simulink model "ReqsGroundTruth"  (R2021b)
settings: Solver=FixedStepAuto  StartTime=0.0  StopTime=stopTime  RelTol=1e-3
model workspace (MAT data in the model file):
  firstWarning = 1
  originalScenarioChecksum = '114339432DE22364D47BB28FC96DC10C'
undefined symbols (not defined in the file): Acceleration, ActorID, AngularVelocity, DefaultGear, DEND_B, DEND_S, DEND_T, LF, LR, MAX_BRAKE, MAX_STEER, MAX_TORQUE, MCAR, MIN_BRAKE, MIN_STEER, MIN_TORQUE, NUMD_B, NUMD_S, NUMD_T, Pitch, Position, R, Roll, RRdamp, scenario, sigbuilder_block, STEER_RATIO, stopSign_ID, Tdead, TL_ID, TrackWidth, Ts, ts, Vdead, Velocity, X_o, Y_o, Yaw
libraries: sim3dprobsensorlib x2, sim3dcameralib x2, drivingscenarioandsensors x2, simulink x1, mspsensorlib x1, sim3dphyssensorlib x1, autolibshared x1, vehdynlibviscommon x1, vehdynlibsteering x1
settings Model: SimulationMode=software-in-the-loop (sil)  Creator=akshran  LastModifiedBy=akshran
settings OptimizationCC: DefaultParameterBehavior=Inlined  EnhancedBackFolding=on  PassReuseOutputArgsAs=Individual arguments  ZeroExternalMemoryAtStartup=off  ZeroInternalMemoryAtStartup=off  OptimizeBlockOrder=speed  DifferentSizesBufferReuse=on  OptimizationCustomize=off  EfficientTunableParamExpr=on
settings DebuggingCC: ParameterTunabilityLossMsg=error
settings SFSimCC: MATLABDynamicMemAlloc=off
settings RTWCC: Description=Embedded Coder  SystemTargetFile=ert.tlc  TemplateMakefile=ert_default_tmf  BuildConfiguration=Faster Runs  CodeExecutionProfiling=on  CodeProfilingSaveOptions=AllData  TargetLang=C++
settings CodeAppCC: ForceParamTrailComments=on  IgnoreCustomStorageClasses=off  OperatorAnnotations=on  SimulinkDataObjDesc=on  SFDataObjDesc=on  InsertBlockDesc=on
settings ERTTargetCC: TargetLangStandard=C++11 (ISO)  GenerateSampleERTMain=on  CodeInterfacePackaging=C++ class  SupportContinuousTime=on  SupportVariableSizeSignals=on  InlinedParameterPlacement=NonHierarchical  RootIOFormat=Structure reference  ERTCustomFileTemplate=example_file_process.tlc
settings ConfigComp: CovEnable=on  CovScope=ReferencedModels  CovIncludeTopModel=off  CovMetricSettings=dtrzoibwe  CovModelRefEnable=filtered

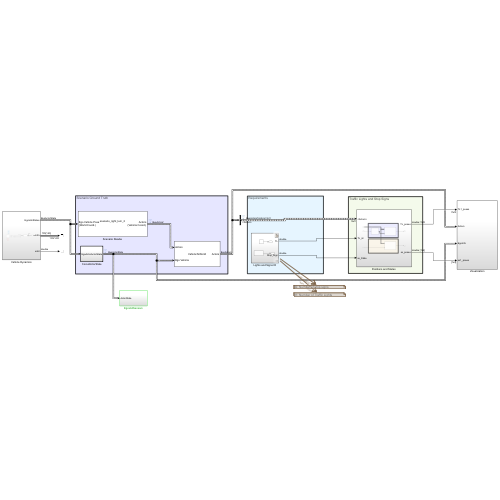
[thumbnail: Simulink's stored preview of the top-level diagram]
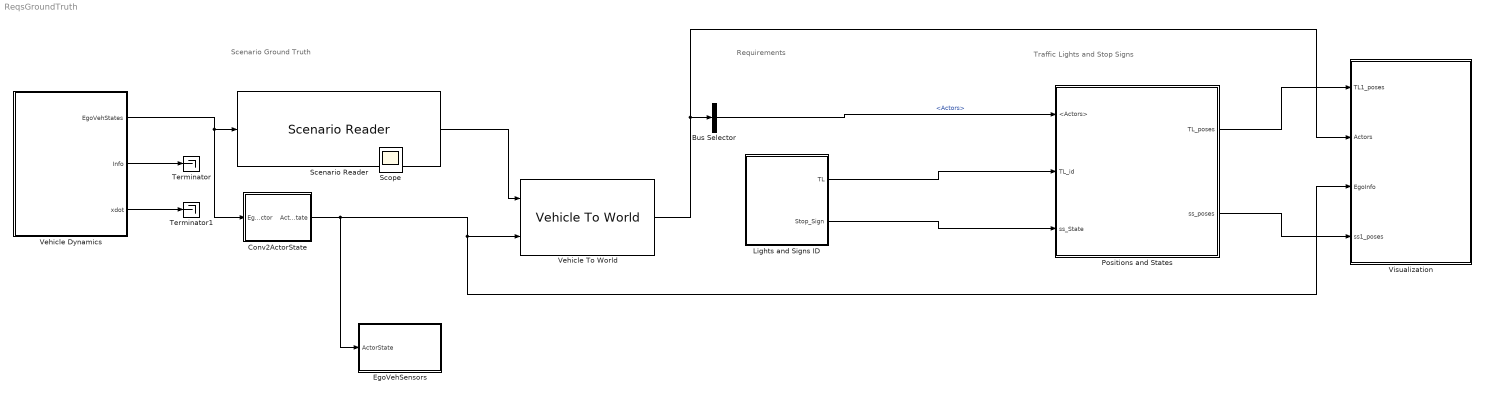
== system ReqsGroundTruth ==
  note: Traffic Lights and Stop Signs
  note: Requirements
  note: Scenario Ground Truth
  Bus Selector : BusSelector  OutputSignals=Actors
  Conv2ActorState : Subsystem  TreatAsAtomicUnit=on
  EgoVehSensors : Subsystem
  Lights and Signs ID : Subsystem
  "Positions and States " : Subsystem
  Scenario Reader : drivingscenarioandsensors/Scenario Reader  ScenarioSource=From file  ScenarioFileName=C:\Users\akshran\MATLAB\Projects\ad2_y1_simulationpkg\scenarios\scenario_right_turn_2.mat  ScenarioVariableName=scenario  OutputCoordinateSystem=Vehicle coordinates  EgoVehicleSource=Input port  EgoVehicleActorID=1  OrientVehiclesOnRoad=on  OutputEgoVehiclePose=on  OutputEgoVehicleState=off  SampleTime=Ts  LaneBoundaryOutput=None  LaneBoundaryDistance=0:0.5:9.5  LaneBoundaryLocation=Center of lane markings  BusNameSource=Auto  BusName=BusActors  BusNumActorsSource=Scenario  BusNumActors=100  BusName2Source=Auto  BusName2=BusLaneBoundaries  BusNumLaneBoundariesSource=Scenario  BusNumLaneBoundaries=10  BusName3Source=Auto  BusName3=BusEgoActor  BusName4Source=Auto  BusName4=BusEgoState  ShowCoordinateLabels=on  SimulateUsing=Interpreted execution
  Terminator : Terminator
  Terminator1 : Terminator
  Vehicle Dynamics : Subsystem
  Vehicle To World : drivingscenarioandsensors/Vehicle To World  BusNameSource=Auto  BusName=BusVehicleToWorldActors  SimulateUsing=Interpreted execution
      settings: SourceProductBaseCode=DR
  Visualization : Subsystem
  Scope : Scope
  wires:
  Vehicle Dynamics/1(EgoVehStates) -> Conv2ActorState/1(EgoActor), Scenario Reader/1
  Scenario Reader/1 -> Vehicle To World/1
  Conv2ActorState/1(ActorState) -> Visualization/3(EgoInfo), Vehicle To World/2, EgoVehSensors/1(ActorState)
  Vehicle To World/1 -> Visualization/2(Actors), Bus Selector/1
  Vehicle Dynamics/2(Info) -> Terminator/1
  Vehicle Dynamics/3(xdot) -> Terminator1/1
  Bus Selector/1 -> "Positions and States "/1(<Actors>)  "<Actors>"
  Lights and Signs ID/1(TL) -> "Positions and States "/2(TL_id)
  Lights and Signs ID/2(Stop_Sign) -> "Positions and States "/3(ss_State)
  "Positions and States "/1(TL_poses) -> Visualization/1(TL1_poses)
  "Positions and States "/2(ss_poses) -> Visualization/4(ss1_poses)

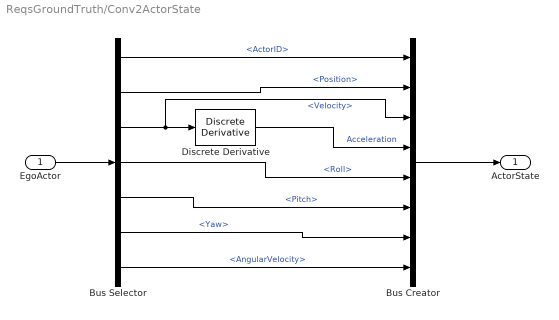
== system ReqsGroundTruth/Conv2ActorState ==
  EgoActor : Inport
  Bus Creator : BusCreator  Inputs=ActorID,Position,Velocity,Acceleration,Roll,Pitch,Yaw,AngularVelocity  OutDataTypeStr=Bus: BusActorState  NonVirtualBus=on
  Bus Selector : BusSelector  OutputSignals=ActorID,Position,Velocity,Roll,Pitch,Yaw,AngularVelocity
  Discrete Derivative : simulink/Discrete/Discrete Derivative  gainval=1.0  ICPrevScaledInput=0.0  OutMin=[]  OutMax=[]  OutDataType=fixdt(1, 16)  OutScaling=2^-10  DoSatur=off
  ActorState : Outport
  wires:
  Bus Selector/3 -> Bus Creator/3, Discrete Derivative/1  "<Velocity>"
  Bus Selector/2 -> Bus Creator/2  "<Position>"
  Bus Selector/7 -> Bus Creator/8  "<AngularVelocity>"
  Discrete Derivative/1 -> Bus Creator/4  "Acceleration"
  Bus Selector/1 -> Bus Creator/1  "<ActorID>"
  Bus Selector/6 -> Bus Creator/7  "<Yaw>"
  Bus Selector/5 -> Bus Creator/6  "<Pitch>"
  Bus Selector/4 -> Bus Creator/5  "<Roll>"
  EgoActor/1 -> Bus Selector/1
  Bus Creator/1 -> ActorState/1

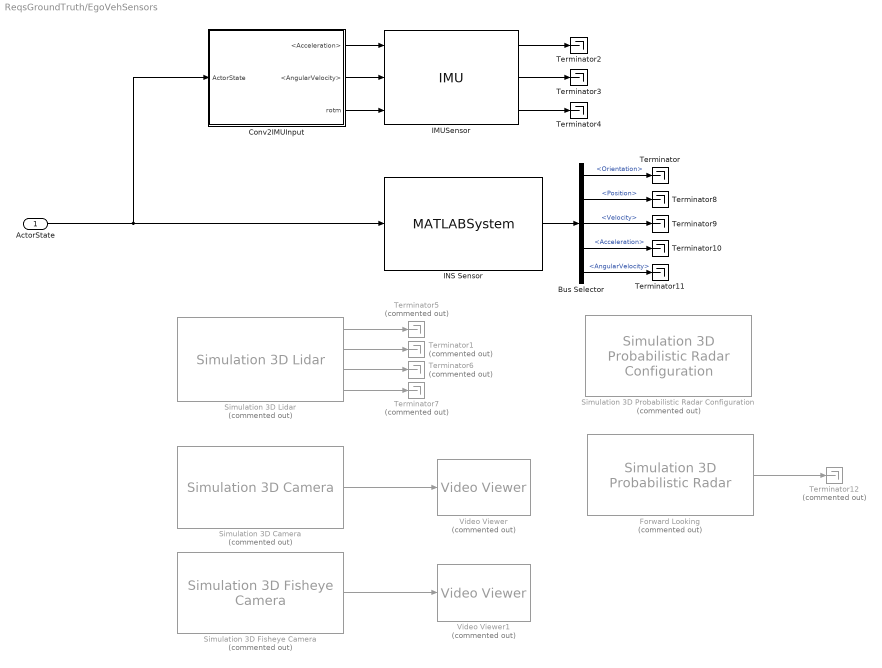
== system ReqsGroundTruth/EgoVehSensors ==
  ActorState : Inport
  Bus Selector : BusSelector  OutputSignals=Orientation,Position,Velocity,Acceleration,AngularVelocity
  Conv2IMUInput : Subsystem  TreatAsAtomicUnit=on
  Forward Looking : sim3dprobsensorlib/Simulation 3D Probabilistic Radar  Priority=1  Commented=on  sensorTag=Sim3dSensor1  sensorId=1  sensorName=Sim3dSensor1  vehTagList={'Scene Origin'}  vehTag=Scene Origin  mountLoc=Origin  offsetFlag=off  tmountOffset=[0, 0, 0]  rmountOffset=[0, 0, 0]  AzimuthResolution=4  ElevationResolution=10  RangeResolution=2.5  RangeRateResolution=0.5  AzimuthBiasFraction=0.1  ElevationBiasFraction=0.1  RangeBiasFraction=0.05  RangeRateBiasFraction=0.05  FieldOfView=[ 45, 5 ]  DetectionRange=[ 1, 150 ]  RangeRateLimits=[ -100, 100 ]  DetectionProbability=0.9  FalseAlarmRate=1e-6  ReferenceRange=100  ReferenceRCS=0  HasElevation=off  HasRangeRate=on  HasNoise=on  HasFalseAlarms=on  InitialSeedSource=Repeatable  InitialSeed=0  MaxNumDetections=50  DetectionCoordinates=Ego Cartesian  SpecifyOutputBusName=off  BusName=BusSimulation3DRadarTruthSensor  SampleTime=-1  mountPoint=[0 0 0]  mountOrientation=[0 0 0]  aMode=3  ID=1
      settings: SourceProductBaseCode=AE,DR,UV,VE
  IMUSensor : mspsensorlib/IMU  DispRefFrame=NED  Temperature=25  MagneticFieldNED=[ 27.5550, -2.4169, -16.0849 ]  MagneticFieldENU=[ -2.4169, 27.5550, 16.0849 ]  SeedDouble=67  SimulateUsing=Interpreted execution  AccelParamsMeasurementRange=Inf  AccelParamsResolution=0  AccelParamsConstantBias=[ 0, 0, 0 ]  AccelParamsAxesMisalignment=[ 0, 0, 0 ]  AccelParamsNoiseDensity=[ 0, 0, 0 ]  AccelParamsBiasInstability=[ 0, 0, 0 ]  AccelParamsRandomWalk=[ 0, 0, 0 ]  AccelParamsTemperatureBias=[ 0, 0, 0 ]  AccelParamsTemperatureScaleFactor=[ 0, 0, 0 ]  GyroParamsMeasurementRange=Inf  GyroParamsResolution=0  GyroParamsConstantBias=[ 0, 0, 0 ]  GyroParamsAxesMisalignment=[ 0, 0, 0 ]  GyroParamsAccelerationBias=[ 0, 0, 0 ]  GyroParamsNoiseDensity=[ 0, 0, 0 ]  GyroParamsBiasInstability=[ 0, 0, 0 ]  GyroParamsRandomWalk=[ 0, 0, 0 ]  GyroParamsTemperatureBias=[ 0, 0, 0 ]  GyroParamsTemperatureScaleFactor=[ 0, 0, 0 ]  MagParamsMeasurementRange=Inf  MagParamsResolution=0  MagParamsConstantBias=[ 0, 0, 0 ]  MagParamsAxesMisalignment=[ 0, 0, 0 ]  MagParamsNoiseDensity=[ 0, 0, 0 ]  MagParamsBiasInstability=[ 0, 0, 0 ]  MagParamsRandomWalk=[ 0, 0, 0 ]  MagParamsTemperatureBias=[ 0, 0, 0 ]  MagParamsTemperatureScaleFactor=[ 0, 0, 0 ]
      settings: SourceProductBaseCode=TF,NV
  INS Sensor : MATLABSystem  System=insSensorBlk  MountingLocation=[ 0, 0, 0 ]  RollAccuracy=0.2  PitchAccuracy=0.2  YawAccuracy=1  PositionAccuracy=[ 1, 1, 1 ]  VelocityAccuracy=0.1  AccelerationAccuracy=0.05  AngularVelocityAccuracy=0.5  PositionErrorFactor=[ 0, 0, 0 ]  OutputBusName1=BusINSMeas  SimulateUsing=Interpreted execution
      mask Type: insSensorBlk
      mask Display:
      | disp('insSensorBlk');
      | port_label('input',1,'ActorStateIn');
      | port_label('output',1,'insMeas');
  Simulation 3D Camera : sim3dcameralib/Simulation 3D Camera  Priority=1  Commented=on  sensorTag=Sim3dSensor2  sensorId=2  sensorName=Sim3dSensor2  vehTagList={'Scene Origin'}  vehTag=Scene Origin  mountLoc=Origin  offsetFlag=off  tmountOffset=[0, 0, 0]  extTmount=off  rmountOffset=[0, 0, 0]  extRmount=off  FocalLength=[1109, 1109]  OpticalCenter=[640, 360]  ImageSize=[720, 1280]  RadialDistortion=[0, 0]  TangentialDistortion=[0, 0]  SensorSkew=0  DepthOutportEnabled=off  SemanticOutportEnabled=off  TransformOutportEnabled=off  SampleTime=-1  mountPoint=[0 0 0]  mountOrientation=[0 0 0]  aMode=3  ID=2
      settings: SourceProductBaseCode=AE,DR,UV,VE
  Simulation 3D Fisheye Camera : sim3dcameralib/Simulation 3D Fisheye Camera  Priority=1  Commented=on  sensorTag=Sim3dSensor3  sensorId=3  sensorName=Sim3dSensor3  vehTagList={'Scene Origin'}  vehTag=Scene Origin  mountLoc=Origin  offsetFlag=off  tmountOffset=[0, 0, 0]  extTmount=off  rmountOffset=[0, 0, 0]  extRmount=off  OpticalCenter=[640, 360]  ImageSize=[720, 1280]  RadialDistortion=[320, 0, 0, 0]  StretchMatrix=[1, 0; 0, 1]  TransformOutportEnabled=off  SampleTime=-1  mountPoint=[0 0 0]  mountOrientation=[0 0 0]  aMode=3  ID=3
      settings: SourceProductBaseCode=AE,DR,UV,VE
  Simulation 3D Lidar : sim3dphyssensorlib/Simulation 3D Lidar  Priority=1  Commented=on  sensorTag=Sim3dSensor4  sensorId=4  sensorName=Sim3dSensor4  vehTagList={'Scene Origin'}  vehTag=Scene Origin  mountLoc=Origin  offsetFlag=off  tmountOffset=[0, 0, 0]  rmountOffset=[0, 0, 0]  DetectionRange=120  RangeResolution=0.002  VerticalFOV=40  VerticalResolution=1.25  HorizontalFOV=360  HorizontalResolution=0.16  DistanceOutportEnabled=on  TransformOutportEnabled=on  SampleTime=0.05  mountPoint=[0 0 0]  mountOrientation=[0 0 0]  aMode=3  ID=4
      settings: SourceProductBaseCode=AE,DR,UV,VE
  Simulation 3D Probabilistic Radar Configuration : sim3dprobsensorlib/Simulation 3D Probabilistic Radar Configuration  Commented=on  RCSactorKeys=[10]  RCSactorProfiles={[10, 10;10, 10]}  RCSdefaultValue=-20  aMode=3
      settings: SourceProductBaseCode=AE,DR,UV,VE
  Terminator{,2..4,8..11} (8 alike) : Terminator
  Terminator{1,5..7,12} (5 alike) : Terminator  Commented=on
  Video Viewer : VideoViewer  Commented=on  FigPos=[1958 858 1025 616]
  Video Viewer1 : VideoViewer  Commented=on  FigPos=[2014 821 1025 616]
  wires:
  ActorState/1 -> INS Sensor/1, Conv2IMUInput/1(ActorState)
  INS Sensor/1 -> Bus Selector/1
  IMUSensor/1 -> Terminator2/1
  IMUSensor/2 -> Terminator3/1
  IMUSensor/3 -> Terminator4/1
  Conv2IMUInput/1(<Acceleration>) -> IMUSensor/1
  Conv2IMUInput/2(<AngularVelocity>) -> IMUSensor/2
  Conv2IMUInput/3(rotm) -> IMUSensor/3
  Simulation 3D Lidar/1 -> Terminator5/1
  Simulation 3D Camera/1 -> Video Viewer/1
  Simulation 3D Lidar/2 -> Terminator1/1
  Simulation 3D Lidar/3 -> Terminator6/1
  Simulation 3D Lidar/4 -> Terminator7/1
  Simulation 3D Fisheye Camera/1 -> Video Viewer1/1
  Bus Selector/1 -> Terminator/1  "<Orientation>"
  Bus Selector/2 -> Terminator8/1  "<Position>"
  Bus Selector/3 -> Terminator9/1  "<Velocity>"
  Bus Selector/4 -> Terminator10/1  "<Acceleration>"
  Bus Selector/5 -> Terminator11/1  "<AngularVelocity>"
  Forward Looking/1 -> Terminator12/1

== system ReqsGroundTruth/Lights and Signs ID ==
  Constant : Constant  Value=TL_ID
  Constant1 : Constant  Value=stopSign_ID
  TL : Outport
  Stop_Sign : Outport  Port=2
  wires:
  Constant/1 -> TL/1
  Constant1/1 -> Stop_Sign/1

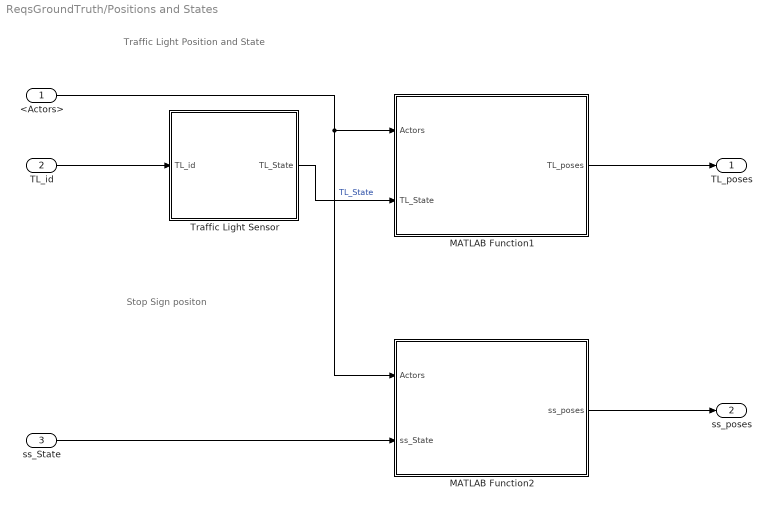
== system ReqsGroundTruth/Positions and States  ==
  note: Stop Sign positon
  note: Traffic Light Position and State
  <Actors> : Inport
  TL_id : Inport  Port=2
  ss_State : Inport  Port=3
  MATLAB Function1 : MATLAB Function  TreatAsAtomicUnit=on
  MATLAB Function2 : MATLAB Function  TreatAsAtomicUnit=on
  Traffic Light Sensor : Subsystem  mask{TrafficLightSensorModeSelection=Cycle}
      mask prompts: TrafficLightSensorModeSelection "Traffic Light Sensor Mode:"
      mask TypeOptions TrafficLightSensorModeSelection: Steady Green | Steady Red | Cycle
      mask DialogControl DescTextVar Prompt: Simulate a traffic light sensor.
  TL_poses : Outport
  ss_poses : Outport  Port=2
  wires:
  <Actors>/1 -> MATLAB Function2/1(Actors), MATLAB Function1/1(Actors)
  ss_State/1 -> MATLAB Function2/2(ss_State)
  TL_id/1 -> Traffic Light Sensor/1(TL_id)
  Traffic Light Sensor/1(TL_State) -> MATLAB Function1/2(TL_State)  "TL_State"
  MATLAB Function2/1(ss_poses) -> ss_poses/1
  MATLAB Function1/1(TL_poses) -> TL_poses/1

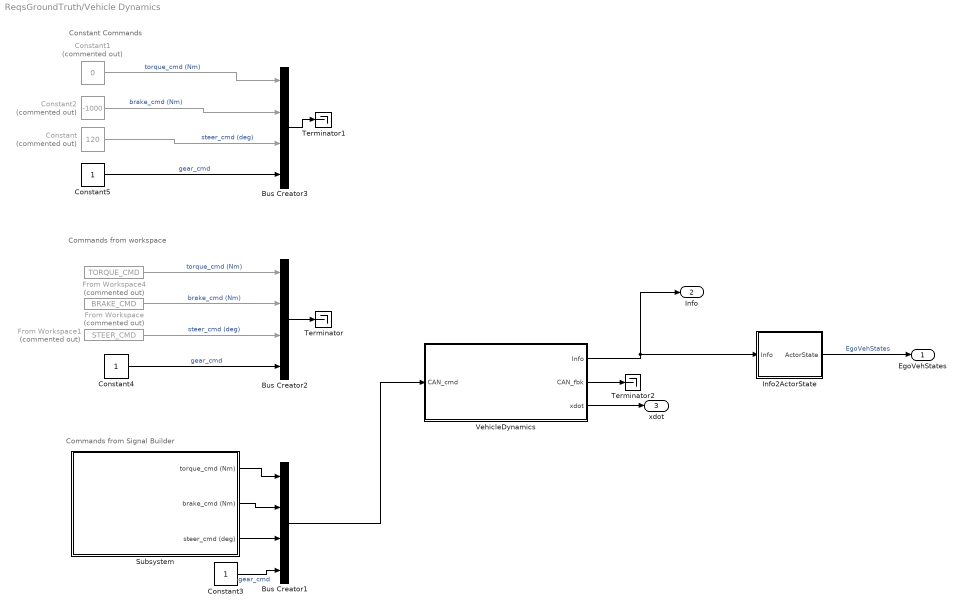
== system ReqsGroundTruth/Vehicle Dynamics ==
  note: Constant Commands
  note: Commands from workspace
  note: Commands from Signal Builder
  Bus Creator1 : BusCreator  Inputs=4
  Bus Creator2 : BusCreator  Inputs=4
  Bus Creator3 : BusCreator  Inputs=4
  Constant : Constant  Commented=on  Value=120
  Constant1 : Constant  Commented=on  Value=0
  Constant2 : Constant  Commented=on  Value=-1000
  Constant3 : Constant
  Constant4 : Constant
  Constant5 : Constant
  From Workspace : FromWorkspace  Commented=on  VariableName=BRAKE_CMD  SampleTime=ts
  From Workspace1 : FromWorkspace  Commented=on  VariableName=STEER_CMD  SampleTime=ts
  From Workspace4 : FromWorkspace  Commented=on  VariableName=TORQUE_CMD  SampleTime=ts
  Info2ActorState : Subsystem
  Subsystem : Subsystem
  Terminator : Terminator
  Terminator1 : Terminator
  Terminator2 : Terminator
  VehicleDynamics : Subsystem  mask{InitPosition=scenario.Actors(1).Position-0.5*scenario.Actors(1).Wheelbase*[cosd(scenario.Actors(1).Yaw) sind(scenario.Actors(1).Yaw) 0], InitSpeed=norm(scenario.Actors(1).Velocity), InitYaw=scenario.Actors(1).Yaw}
      mask prompts: InitPosition "Initial Position (m)"; InitSpeed "Initial Speed (m/s)"; InitYaw "Init Yaw (rad)"
  EgoVehStates : Outport
  Info : Outport  Port=2
  xdot : Outport  Port=3
  wires:
  Bus Creator2/1 -> Terminator/1
  VehicleDynamics/2(CAN_fbk) -> Terminator2/1
  VehicleDynamics/1(Info) -> Info/1, Info2ActorState/1(Info)
  Constant/1 -> Bus Creator3/3  "steer_cmd (deg)"
  Info2ActorState/1(ActorState) -> EgoVehStates/1  "EgoVehStates"
  Constant1/1 -> Bus Creator3/1  "torque_cmd (Nm)"
  Constant2/1 -> Bus Creator3/2  "brake_cmd (Nm)"
  VehicleDynamics/3(xdot) -> xdot/1
  Subsystem/1(torque_cmd (Nm)) -> Bus Creator1/1
  Subsystem/2(brake_cmd (Nm)) -> Bus Creator1/2
  Subsystem/3(steer_cmd (deg)) -> Bus Creator1/3
  Constant3/1 -> Bus Creator1/4  "gear_cmd"
  Bus Creator1/1 -> VehicleDynamics/1(CAN_cmd)
  Constant4/1 -> Bus Creator2/4  "gear_cmd"
  From Workspace/1 -> Bus Creator2/2  "brake_cmd (Nm)"
  From Workspace1/1 -> Bus Creator2/3  "steer_cmd (deg)"
  From Workspace4/1 -> Bus Creator2/1  "torque_cmd (Nm)"
  Constant5/1 -> Bus Creator3/4  "gear_cmd"
  Bus Creator3/1 -> Terminator1/1

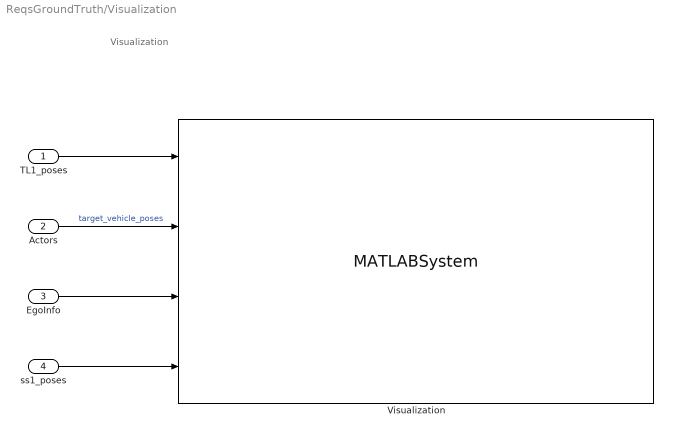
== system ReqsGroundTruth/Visualization ==
  note: Visualization
  TL1_poses : Inport
  Actors : Inport  Port=2
  EgoInfo : Inport  Port=3
  ss1_poses : Inport  Port=4
  Visualization : MATLABSystem  System=TL_vis
      mask Type: TL_vis
      mask Display:
      | disp('TL_vis');
      | port_label('input',1,'TL');
      | port_label('input',2,'TargetPoses');
      | port_label('input',3,'EgoInfo');
      | port_label('input',4,'SS');
  wires:
  EgoInfo/1 -> Visualization/3
  Actors/1 -> Visualization/2  "target_vehicle_poses"
  TL1_poses/1 -> Visualization/1
  ss1_poses/1 -> Visualization/4

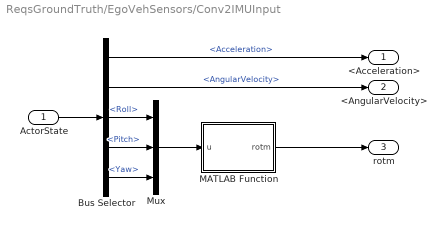
== system ReqsGroundTruth/EgoVehSensors/Conv2IMUInput ==
  ActorState : Inport
  Bus Selector : BusSelector  OutputSignals=Acceleration,AngularVelocity,Roll,Pitch,Yaw
  MATLAB Function : MATLAB Function  TreatAsAtomicUnit=on
  Mux : Mux  Inputs=3
  <Acceleration> : Outport
  <AngularVelocity> : Outport  Port=2
  rotm : Outport  Port=3
  wires:
  Bus Selector/4 -> Mux/2  "<Pitch>"
  Bus Selector/3 -> Mux/1  "<Roll>"
  ActorState/1 -> Bus Selector/1
  MATLAB Function/1(rotm) -> rotm/1
  Mux/1 -> MATLAB Function/1(u)
  Bus Selector/2 -> <AngularVelocity>/1  "<AngularVelocity>"
  Bus Selector/5 -> Mux/3  "<Yaw>"
  Bus Selector/1 -> <Acceleration>/1  "<Acceleration>"

== system ReqsGroundTruth/Positions and States /Traffic Light Sensor ==
  note: Traffic Light Sensor
  TL_id : Inport
  Bus Creator : BusCreator  Inputs=2
  LightConfiguration : Constant  Value=TrafficLightSensorModeSelection
  Traffic Light Switching Logic : Stateflow chart  TreatAsAtomicUnit=on
  TL_State : Outport
  wires:
  LightConfiguration/1 -> Traffic Light Switching Logic/1(LightConfig)
  TL_id/1 -> Traffic Light Switching Logic/2(TL_id)
  Bus Creator/1 -> TL_State/1
  Traffic Light Switching Logic/2(trafficLight) -> Bus Creator/1
  Traffic Light Switching Logic/1(TL_ID) -> Bus Creator/2

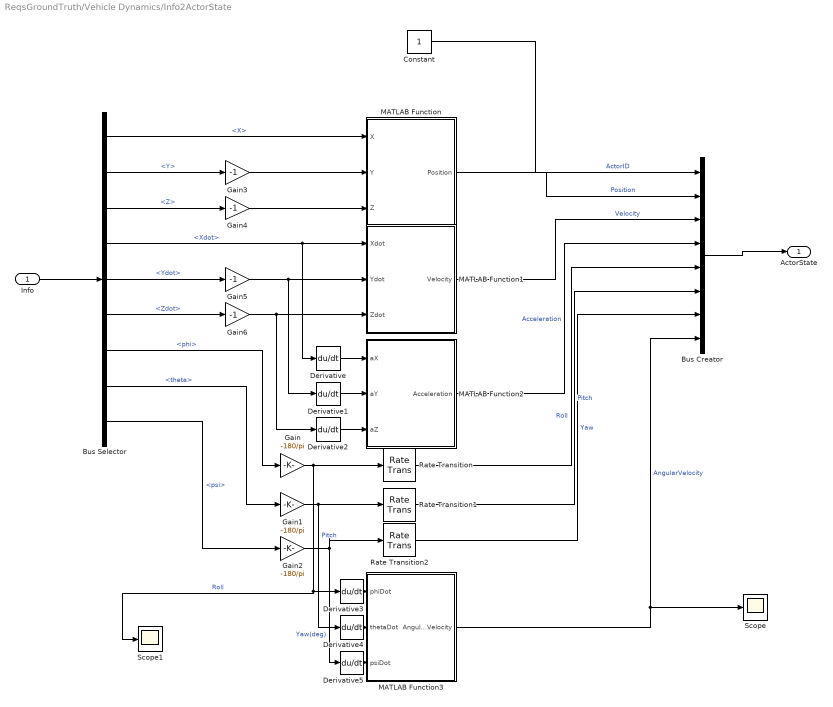
== system ReqsGroundTruth/Vehicle Dynamics/Info2ActorState ==
  Info : Inport
  Bus Creator : BusCreator  Inputs=ActorID,Position,Velocity,Acceleration,Roll,Pitch,Yaw,AngularVelocity  OutDataTypeStr=Bus: BusActorState  NonVirtualBus=on
  Bus Selector : BusSelector  OutputSignals=InertFrm.Cg.Disp.X,InertFrm.Cg.Disp.Y,InertFrm.Cg.Disp.Z,InertFrm.Cg.Vel.Xdot,InertFrm.Cg.Vel.Ydot,InertFrm.Cg.Vel.Zdot,InertFrm.Cg.Ang.phi,InertFrm.Cg.Ang.theta,InertFrm.Cg.Ang.psi
  Constant : Constant  SampleTime=0.05
  Derivative{,1..5} (6 alike) : Derivative
  Gain : Gain  Gain=-180/pi
  Gain1 : Gain  Gain=-180/pi
  Gain2 : Gain  Gain=-180/pi
  Gain{3..6} (4 alike) : Gain  Gain=-1
  MATLAB Function : MATLAB Function  TreatAsAtomicUnit=on  SystemSampleTime=0.05
  MATLAB Function1 : MATLAB Function  TreatAsAtomicUnit=on  SystemSampleTime=0.05
  MATLAB Function2 : MATLAB Function  TreatAsAtomicUnit=on  SystemSampleTime=0.05
  MATLAB Function3 : MATLAB Function  TreatAsAtomicUnit=on  SystemSampleTime=0.05
  Rate Transition : RateTransition  OutPortSampleTime=0.05
  Rate Transition1 : RateTransition  OutPortSampleTime=0.05
  Rate Transition2 : RateTransition  OutPortSampleTime=0.05
  Scope : Scope
  Scope1 : Scope
  ActorState : Outport
  wires:
  Gain/1 -> Scope1/1, Derivative3/1, Rate Transition/1  "Roll"
  Derivative4/1 -> MATLAB Function3/2(thetaDot)
  Bus Selector/2 -> Gain3/1  "<Y>"
  Bus Selector/4 -> Derivative/1, MATLAB Function1/1(Xdot)  "<Xdot>"
  MATLAB Function1/1(Velocity) -> Bus Creator/3  "Velocity"
  MATLAB Function/1(Position) -> Bus Creator/2  "Position"
  Derivative1/1 -> MATLAB Function2/2(aY)
  Bus Selector/5 -> Gain5/1  "<Ydot>"
  Bus Selector/1 -> MATLAB Function/1(X)  "<X>"
  Bus Selector/9 -> Gain2/1  "<psi>"
  Gain2/1 -> Rate Transition2/1, Derivative5/1  "Yaw(deg)"
  Derivative5/1 -> MATLAB Function3/3(psiDot)
  Bus Selector/7 -> Gain/1  "<phi>"
  MATLAB Function2/1(Acceleration) -> Bus Creator/4  "Acceleration"
  Derivative3/1 -> MATLAB Function3/1(phiDot)
  Gain1/1 -> Derivative4/1, Rate Transition1/1  "Pitch"
  Bus Selector/6 -> Gain6/1  "<Zdot>"
  Bus Selector/8 -> Gain1/1  "<theta>"
  MATLAB Function3/1(AngularVelocity) -> Bus Creator/8, Scope/1  "AngularVelocity"
  Bus Selector/3 -> Gain4/1  "<Z>"
  Derivative2/1 -> MATLAB Function2/3(aZ)
  Derivative/1 -> MATLAB Function2/1(aX)
  Info/1 -> Bus Selector/1
  Constant/1 -> Bus Creator/1  "ActorID"
  Bus Creator/1 -> ActorState/1
  Rate Transition/1 -> Bus Creator/5  "Roll"
  Rate Transition1/1 -> Bus Creator/6  "Pitch"
  Rate Transition2/1 -> Bus Creator/7  "Yaw"
  Gain3/1 -> MATLAB Function/2(Y)
  Gain4/1 -> MATLAB Function/3(Z)
  Gain5/1 -> Derivative1/1, MATLAB Function1/2(Ydot)
  Gain6/1 -> Derivative2/1, MATLAB Function1/3(Zdot)

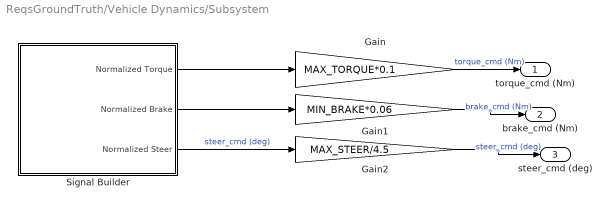
== system ReqsGroundTruth/Vehicle Dynamics/Subsystem ==
  Gain : Gain  Gain=MAX_TORQUE*0.1
  Gain1 : Gain  Gain=MIN_BRAKE*0.06
  Gain2 : Gain  Gain=MAX_STEER/4.5
  Signal Builder : Subsystem  Tag=STV Subsys  LoadFcn=sigbuilder_block('load');  StartFcn=sigbuilder_block('start');  StopFcn=sigbuilder_block('stop');  ClipboardFcn=sigbuilder_block('clipboard');  mask(Sigbuilder block){tuvar=[0:10]}
      mask help: Simulink:masks:SigbuilderBlock_MD
      mask init:
      | if ~strcmp(get_param(bdroot(gcbh),'SimulationStatus'),'stopped') tuvar = sigbuilder_block('maskInit'); end
      settings: CopyFcn=sigbuilder_block('copy');  DeleteFcn=sigbuilder_block('delete');  ModelCloseFcn=sigbuilder_block('modelClose');  PreSaveFcn=sigbuilder_block('preSave');  PauseFcn=sigbuilder_block('pause');  ContinueFcn=sigbuilder_block('continue');  NameChangeFcn=sigbuilder_block('namechange');  OpenFcn=sigbuilder_block('open',[0 30 960 455.5 ]);  CloseFcn=sigbuilder_block('close');
      mask Display: plot(0, 0, 100, 100,[2, 2, 32, 32, 2], [68, 8, 8, 68, 68],[32, 2], [38, 38], [32, 19, 2],[53, 60, 44], [32, 17, 17, 2],[16, 16, 31, 31]);txt = getActiveGroup(gcbh);text(2, 100, txt,'verticalAlignment', 'top');
  torque_cmd (Nm) : Outport
  brake_cmd (Nm) : Outport  Port=2
  steer_cmd (deg) : Outport  Port=3
  wires:
  Gain2/1 -> steer_cmd (deg)/1  "steer_cmd (deg)"
  Signal Builder/1(Normalized Torque) -> Gain/1
  Signal Builder/2(Normalized Brake) -> Gain1/1
  Signal Builder/3(Normalized Steer) -> Gain2/1  "steer_cmd (deg)"
  Gain1/1 -> brake_cmd (Nm)/1  "brake_cmd (Nm)"
  Gain/1 -> torque_cmd (Nm)/1  "torque_cmd (Nm)"

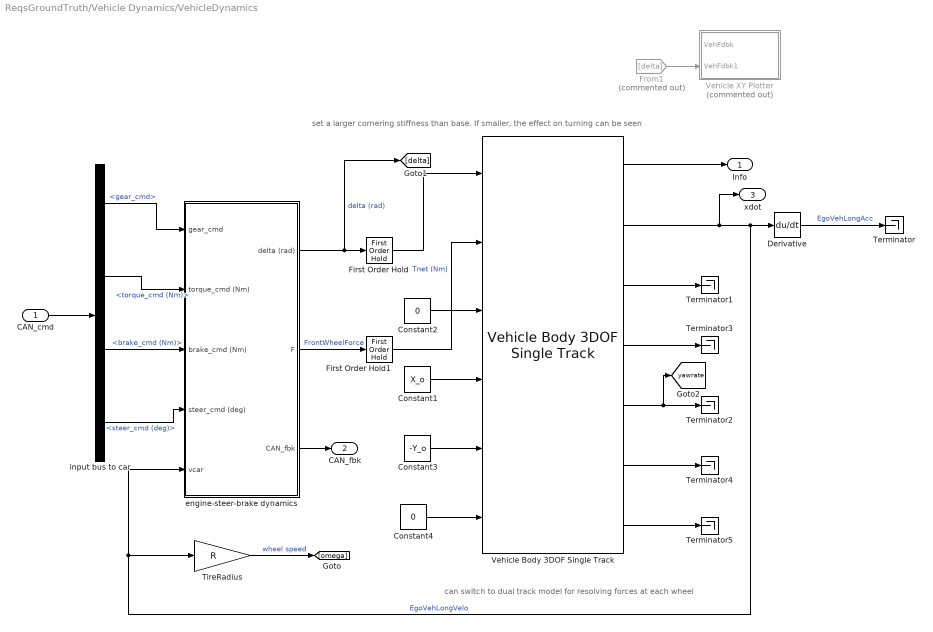
== system ReqsGroundTruth/Vehicle Dynamics/VehicleDynamics ==
  note: set a larger cornering stiffness than base. If smaller, the effect on turning can be seen
  note: can switch to dual track model for resolving forces at each wheel
  CAN_cmd : Inport
  Constant1 : Constant  Value=X_o
  Constant2 : Constant  Value=0
  Constant3 : Constant  Value=-Y_o
  Constant4 : Constant  Value=0
  Derivative : Derivative
  First Order Hold : FirstOrderHold  ErrorTolerance=inf
  First Order Hold1 : FirstOrderHold  ErrorTolerance=inf
  From1 : From  Commented=on  GotoTag=delta
  Terminator{,1..5} (6 alike) : Terminator
  TireRadius : Gain  Gain=R
  Vehicle Body 3DOF Single Track : autolibshared/Vehicle Body 3DOF Single Track  trackMode=Single (bicycle)  inputMode=External longitudinal forces  frontSteerMode=on  rearSteerMode=off  windMode=off  muMode=off  extFMode=off  extMMode=off  htchFMode=off  htchMMode=off  extXo=on  extpsio=on  extxdoto=off  extro=off  extYo=on  extTamb=off  extydoto=off  aMode=2  NF=2  NR=2  m=MCAR  a=LF  b=LR  h=0.35  dh=1  hh=0.2  X_o=InitPosition(1)  xdot_o=InitSpeed  CalphaMode=off  sigmaMode=on  d=0  hl=0  w=[1.4,1.4]  Cy_f=12e3*100  Cy_r=11e3*100  sigma_f=.1  sigma_r=.1  alpha_f_brk=[-.1 .1]  Cy_f_data=[-9e3 9e3]  alpha_r_brk=[-.1 .1]  Cy_r_data=[-9e3 9e3]  Y_o=-InitPosition(2)  ydot_o=0  Izz=2050  psi_o=-InitYaw/180*pi  r_o=0  Af=2  Cd=.3  Cl=.1  Cpm=.1  beta_w=[0:0.01:0.3]  Cs=[0:0.03:0.9]  Cym=[0:0.01:0.3]  Pabs=101325  Tair=273  g=9.81  mu=1  xdot_tol=.01  Fznom=5000  Fxtire_sat=7e4  Fytire_sat=7e4  longOff=0  latOff=0  vertOff=0  wrapAng=off
      settings: SourceProductBaseCode=PW,DR,MT,UV,VE
  Vehicle XY Plotter : Subsystem  Commented=on  mask(Vehicle XY Plotter){a=LF, b=LR, w=TrackWidth, bufferSize=1024, pltDT=.1}
      mask prompts: a "Distance to front axle from CG, a [m]:"; b "Distance to rear axle from CG, b [m]:"; w "Track width, w [m]:"; bufferSize "Path buffer sampe size, bufferSize []:"; pltDT "Plot update rate, pltDT [s]:"
      mask help: This block will display a MATLAB figure which indicates the vehicle path, current position and heading velocity.
      mask TypeOptions a: Vehicle XY Plotter/a
      mask TypeOptions b: Vehicle XY Plotter/b
      mask TypeOptions w: Vehicle XY Plotter/w
      mask TypeOptions bufferSize: Vehicle XY Plotter/bufferSize
  engine-steer-brake dynamics : Subsystem
  input bus to car : BusSelector  OutputSignals=gear_cmd,torque_cmd (Nm),brake_cmd (Nm),steer_cmd (deg)
  Info : Outport
  CAN_fbk : Outport  Port=2  VectorParamsAs1DForOutWhenUnconnected=off
  xdot : Outport  Port=3
  tag scope: yawrate=global
  wires:
  TireRadius/1 -> [omega]  "wheel speed"
  Vehicle Body 3DOF Single Track/1 -> Info/1
  From1/1 -> Vehicle XY Plotter/2(VehFdbk1)
  input bus to car/1 -> engine-steer-brake dynamics/1(gear_cmd)  "<gear_cmd>"
  input bus to car/3 -> engine-steer-brake dynamics/3(brake_cmd (Nm))  "<brake_cmd (Nm)>"
  engine-steer-brake dynamics/1(delta (rad)) -> [delta], First Order Hold/1  "delta (rad)"
  input bus to car/2 -> engine-steer-brake dynamics/2(torque_cmd (Nm))  "<torque_cmd (Nm)>"
  input bus to car/4 -> engine-steer-brake dynamics/4(steer_cmd (deg))  "<steer_cmd (deg)>"
  engine-steer-brake dynamics/3(CAN_fbk) -> CAN_fbk/1
  CAN_cmd/1 -> input bus to car/1
  Constant2/1 -> Vehicle Body 3DOF Single Track/3
  engine-steer-brake dynamics/2(F) -> First Order Hold1/1  "FrontWheelForce"
  First Order Hold/1 -> Vehicle Body 3DOF Single Track/1
  Vehicle Body 3DOF Single Track/2 -> xdot/1, engine-steer-brake dynamics/5(vcar), TireRadius/1, Derivative/1  "EgoVehLongVelo"
  Vehicle Body 3DOF Single Track/3 -> Terminator1/1
  Vehicle Body 3DOF Single Track/4 -> Terminator3/1
  Vehicle Body 3DOF Single Track/5 -> [yawrate], Terminator2/1
  Vehicle Body 3DOF Single Track/6 -> Terminator4/1
  Vehicle Body 3DOF Single Track/7 -> Terminator5/1
  Derivative/1 -> Terminator/1  "EgoVehLongAcc"
  First Order Hold1/1 -> Vehicle Body 3DOF Single Track/2  "Tnet (Nm)"
  Constant1/1 -> Vehicle Body 3DOF Single Track/4
  Constant3/1 -> Vehicle Body 3DOF Single Track/5
  Constant4/1 -> Vehicle Body 3DOF Single Track/6

== system ReqsGroundTruth/Vehicle Dynamics/Subsystem/Signal Builder ==
  Demux : Demux  Tag=STV Demux  Outputs=3
      settings: DisplayOption=none
  FromWs : FromWorkspace  Tag=STV FromWs  VariableName=tuvar
      SigBuilderData=|
      | common.afterFinalStr = 'Extrapolate'
      | common.sampleTime = 0
      | dataSet.timeRange = [0 3.5]
      | dataSet.name = 'DriveAndTurn'
      | sbobj.Groups.Name = 'DriveAndTurn'
      | sbobj.Groups.Signals(1).Name = 'Normalized Torque'
      | sbobj.Groups.Signals(1).XData = [0 1 1 2 2 3.5]
      | sbobj.Groups.Signals(1).YData = [1 1 0 0 1 1]
      | sbobj.Groups.Signals(2).Name = 'Normalized Brake'
      | sbobj.Groups.Signals(2).XData = [0 1 1 2 2 3.5]
      | sbobj.Groups.Signals(2).YData = [0 0 1 1 0 0]
      | sbobj.Groups.Signals(3).Name = 'Normalized Steer'
      | sbobj.Groups.Signals(3).XData = [0 0.5 0.6 1.02 1.02 2 2.5 3 3.5]
      | sbobj.Groups.Signals(3).YData = [-0.02 -0.02 -0.02 -0.3 -1.02 -0.92 -0.34 0.14 0.22]
      | sbobj.Groups.TimeRange = [0 3.5]
  Normalized Torque : Outport  Tag=STV Outport
  Normalized Brake : Outport  Tag=STV Outport  Port=2
  Normalized Steer : Outport  Tag=STV Outport  Port=3
  wires:
  FromWs/1 -> Demux/1
  Demux/1 -> Normalized Torque/1
  Demux/2 -> Normalized Brake/1
  Demux/3 -> Normalized Steer/1

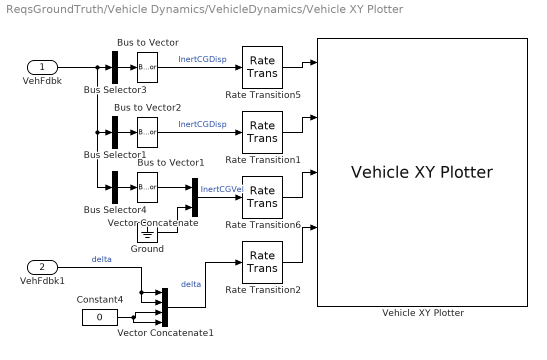
== system ReqsGroundTruth/Vehicle Dynamics/VehicleDynamics/Vehicle XY Plotter ==
  VehFdbk : Inport
  VehFdbk1 : Inport  Port=2
  Bus Selector1 : BusSelector  OutputSignals=InertFrm.Cg.Ang.phi,InertFrm.Cg.Ang.theta,InertFrm.Cg.Ang.psi  OutputAsBus=on
  Bus Selector3 : BusSelector  OutputSignals=InertFrm.Geom.Disp.X,InertFrm.Geom.Disp.Y,InertFrm.Geom.Disp.Z  OutputAsBus=on
  Bus Selector4 : BusSelector  OutputSignals=InertFrm.Cg.Vel.Xdot,InertFrm.Cg.Vel.Ydot  OutputAsBus=on
  Bus to Vector : BusToVector
  Bus to Vector1 : BusToVector
  Bus to Vector2 : BusToVector
  Constant4 : Constant  Value=0
  Ground : Ground
  Rate Transition{1..2,5..6} (4 alike) : RateTransition  OutPortSampleTime=pltDT
  Vector Concatenate : Concatenate
  Vector Concatenate1 : Concatenate  NumInputs=4
  Vehicle XY Plotter : vehdynlibviscommon/Vehicle XY Plotter  w=w  a=a  b=b  figBorder=2000  bufferSize=bufferSize  extStats=off  extTireF=off
      settings: SourceProductName=The database C:\Users\jrodgers\AppData\Roaming\MathWorks\MATLAB\R2018b\slblocks_master.db is locked, or a table in the database is locked. (database is locked)
  wires:
  Bus to Vector2/1 -> Rate Transition1/1  "InertCGDisp"
  Rate Transition5/1 -> Vehicle XY Plotter/1
  Bus Selector4/1 -> Bus to Vector1/1
  Rate Transition1/1 -> Vehicle XY Plotter/2
  Rate Transition6/1 -> Vehicle XY Plotter/3
  Vector Concatenate/1 -> Rate Transition6/1  "InertCGVel"
  Bus Selector1/1 -> Bus to Vector2/1
  Bus to Vector/1 -> Rate Transition5/1  "InertCGDisp"
  Bus Selector3/1 -> Bus to Vector/1
  Bus to Vector1/1 -> Vector Concatenate/1
  Ground/1 -> Vector Concatenate/2
  VehFdbk/1 -> Bus Selector1/1, Bus Selector4/1, Bus Selector3/1
  Rate Transition2/1 -> Vehicle XY Plotter/4
  Constant4/1 -> Vector Concatenate1/4, Vector Concatenate1/3
  VehFdbk1/1 -> Vector Concatenate1/2, Vector Concatenate1/1  "delta"
  Vector Concatenate1/1 -> Rate Transition2/1  "delta"

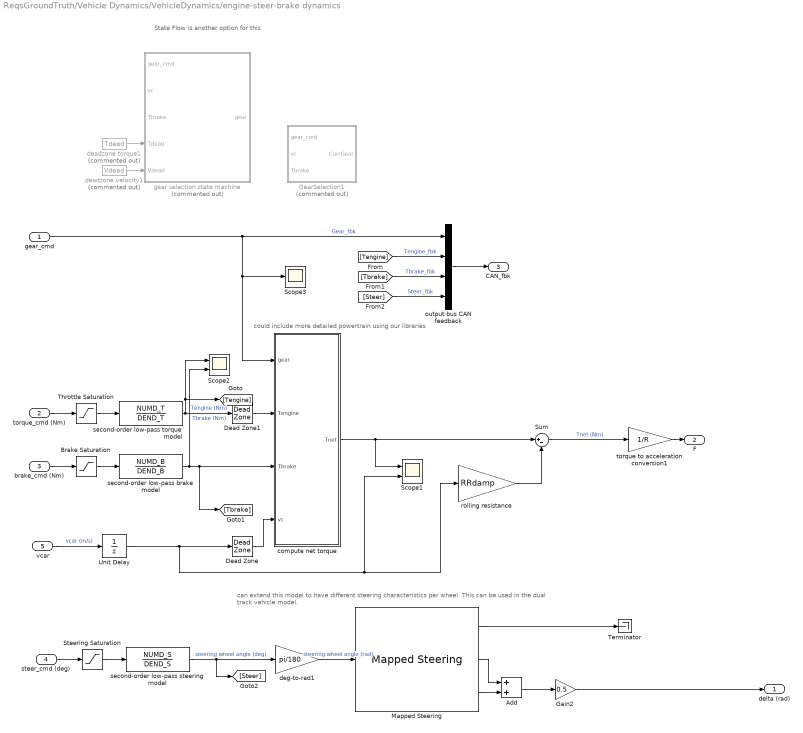
== system ReqsGroundTruth/Vehicle Dynamics/VehicleDynamics/engine-steer-brake dynamics ==
  note: State Flow is another option for this
  note: could include more detailed powertrain using our libraries
  note: can extend this model to have different steering characteristics per wheel. This can be used in the dual track vehicle model.
  gear_cmd : Inport
  torque_cmd (Nm) : Inport  Port=2
  brake_cmd (Nm) : Inport  Port=3
  steer_cmd (deg) : Inport  Port=4
  vcar : Inport  Port=5
  Add : Sum
  Brake Saturation : Saturate  UpperLimit=MAX_BRAKE  LowerLimit=MIN_BRAKE
  Dead Zone : DeadZone  LowerValue=-Vdead  UpperValue=Vdead  SaturateOnIntegerOverflow=on
  Dead Zone1 : DeadZone  LowerValue=-Tdead  UpperValue=Tdead  SaturateOnIntegerOverflow=on
  Gain2 : Gain  Gain=0.5
  GearSelection1 : Stateflow chart  Commented=on  TreatAsAtomicUnit=on  SystemSampleTime=ts
      settings: PortSchema="{\"entries\":[{\"content\":{\"sides\":[{\"content\":{\"connectorIds\":[\"In3\",\"In2\",\"In1\"]},\"type\":\"ConnectorPlacement.EquallySpacedRectSide\",\"uuid\":\"465e5722-891f-481b-b3b6-2b8339e8e743\"},{\"content\":{\"connectorIds\":[\"Out1\"],\"side\":\"RIGHT\"},\"type\":\"ConnectorPlacement.EquallySpacedRectSide\",\"uuid\":\"28ef13cd-41d9-4e2e-8cd9-9157abf573a9\"},{\"content\":{\"connectorIds\":[],\"side\":\"TOP\"},\"type\":\"ConnectorPlacement.EquallySpacedRectSide\",\"uuid\":\"44f19923-60ae-466f-ad2a-756f1033b52e\"},{\"content\":{\"connectorIds\":[],\"side\":\"HIDDEN\"},\"type\":\"ConnectorPlacement.EquallySpacedRectSide\",\"uuid\":\"d5a146f0-4328-42be-94e3-09f51634e7da\"}]},\"type\":\"ConnectorPlacement.EquallySpacedConnector\",\"uuid\":\"14e271af-3da2-4f7d-9688-fcc3c9792006\"}],\"packageUris\":[\"http://schema.mathworks.com/mf0/Connector/R2020b\"],\"version\":\"1.0\"}"
  Mapped Steering : vehdynlibsteering/Mapped Steering  SpdDpd=off  StrgAngBpts=[-1.5*pi 1.5*pi]  WhlLftTbl=[-1.5*pi 1.5*pi]*STEER_RATIO  WhlRghtTbl=[-1.5*pi 1.5*pi]*STEER_RATIO  VehSpdBpts=[-1 1]  SpdFctTbl=[1 1]  aMode=2
      settings: SourceProductBaseCode=VE
  Scope1 : Scope  NumInputPorts=2
  Scope2 : Scope  NumInputPorts=2
  Scope3 : Scope
  Steering Saturation : Saturate  UpperLimit=MAX_STEER  LowerLimit=MIN_STEER
  Sum : Sum  Inputs=|+-
  Terminator : Terminator
  Throttle Saturation : Saturate  UpperLimit=MAX_TORQUE  LowerLimit=MIN_TORQUE
  Unit Delay : UnitDelay  SampleTime=-1  HasFrameUpgradeWarning=on
  compute net torque : MATLAB Function  TreatAsAtomicUnit=on  SystemSampleTime=ts
  deadzone torque1 : Constant  Commented=on  Value=Tdead  SampleTime=ts
  deadzone velocity1 : Constant  Commented=on  Value=Vdead  SampleTime=ts
  deg-to-rad1 : Gain  Gain=pi/180
  gear selection state machine : MATLAB Function  Commented=on  TreatAsAtomicUnit=on  SystemSampleTime=ts
  output bus CAN feedback : BusCreator  Inputs=4
  rolling resistance : Gain  Gain=RRdamp
  second-order low-pass brake model : DiscreteTransferFcn  Numerator=NUMD_B  Denominator=DEND_B  SampleTime=ts
  second-order low-pass steering model : DiscreteTransferFcn  Numerator=NUMD_S  Denominator=DEND_S  SampleTime=ts
  second-order low-pass torque model : DiscreteTransferFcn  Numerator=NUMD_T  Denominator=DEND_T  SampleTime=ts
  torque to acceleration conversion1 : Gain  Gain=1/R
  delta (rad) : Outport  VectorParamsAs1DForOutWhenUnconnected=off
  F : Outport  Port=2  VectorParamsAs1DForOutWhenUnconnected=off
  CAN_fbk : Outport  Port=3  VectorParamsAs1DForOutWhenUnconnected=off
  wires:
  steer_cmd (deg)/1 -> Steering Saturation/1
  torque_cmd (Nm)/1 -> Throttle Saturation/1
  brake_cmd (Nm)/1 -> Brake Saturation/1
  second-order low-pass steering model/1 -> deg-to-rad1/1, [Steer]  "steering wheel angle (deg)"
  Throttle Saturation/1 -> second-order low-pass torque model/1
  Brake Saturation/1 -> second-order low-pass brake model/1
  Steering Saturation/1 -> second-order low-pass steering model/1
  vcar/1 -> Unit Delay/1  "vcar (m/s)"
  second-order low-pass brake model/1 -> [Tbrake], compute net torque/3(Tbrake), Scope2/2  "Tbrake (Nm)"
  second-order low-pass torque model/1 -> Dead Zone1/1, [Tengine], Scope2/1  "Tengine (Nm)"
  compute net torque/1(Tnet) -> Scope1/1, Sum/1
  rolling resistance/1 -> Sum/2
  deadzone velocity1/1 -> gear selection state machine/5(Vdead)
  deadzone torque1/1 -> gear selection state machine/4(Tdead)
  gear_cmd/1 -> output bus CAN feedback/1, Scope3/1, compute net torque/1(gear)  "Gear_fbk"
  output bus CAN feedback/1 -> CAN_fbk/1
  [Tengine] -> output bus CAN feedback/2  "Tengine_fbk"
  [Tbrake] -> output bus CAN feedback/3  "Tbrake_fbk"
  [Steer] -> output bus CAN feedback/4  "Steer_fbk"
  Mapped Steering/2 -> Add/1
  Mapped Steering/3 -> Add/2
  Add/1 -> Gain2/1
  torque to acceleration conversion1/1 -> F/1
  Mapped Steering/1 -> Terminator/1
  deg-to-rad1/1 -> Mapped Steering/1  "steering wheel angle (rad)"
  Sum/1 -> torque to acceleration conversion1/1  "Tnet (Nm)"
  Dead Zone/1 -> compute net torque/4(vc)
  Dead Zone1/1 -> compute net torque/2(Tengine)
  Unit Delay/1 -> Scope1/2, rolling resistance/1, Dead Zone/1
  Gain2/1 -> delta (rad)/1

== stateflow chart ReqsGroundTruth/Vehicle Dynamics/VehicleDynamics/engine-steer-brake dynamics/GearSelection1 ==
  state Park
    CurrGear = 0;
  state Reverse
    CurrGear = -1;
  state drive
    CurrGear = 1;
  (default) -> (junction 12)
  (junction 12) -> Reverse [order 3] : [DefaultGear == -1]
  (junction 12) -> drive [order 2] : [DefaultGear == 1]
  (junction 12) -> Park [order 1] : [DefaultGear == 0]
  (junction 12) -> Park [order 4] : %fallback to park
  drive -> Park [order 2] : [gear_cmd == 0 && allowShift(vc,Tbrake)]
  Park -> Reverse [order 2] : [gear_cmd == -1 && allowShift(vc,Tbrake)]
  Park -> drive [order 1] : [gear_cmd == 1 && allowShift(vc,Tbrake)]
  Reverse -> Park [order 2] : [gear_cmd == 0 && allowShift(vc,Tbrake)]
  drive -> Reverse [order 1] : [gear_cmd == -1 && allowShift(vc,Tbrake)]
  Reverse -> drive [order 1] : [gear_cmd == 1 && allowShift(vc,Tbrake)]
  data: Tdead parameter; Vdead parameter; vel function_input; brakeT function_input; allow function_output; CurrGear output; Tbrake input; vc input; gear_cmd input; DefaultGear parameter
  function allow = allowShift(vel, brakeT):
    | function allow = allowShift(vel, brakeT)
    | allow = (abs(vel) <= Vdead) && (abs(brakeT)>Tdead);
    | end

== matlab function ReqsGroundTruth/EgoVehSensors/Conv2IMUInput/MATLAB Function ==
  data: u input; rotm output size=[3 3]
function rotm = fcn(u)
eul = u/180*pi;
rotm = eul2rotm(eul',"XYZ");
end

== matlab function ReqsGroundTruth/Vehicle Dynamics/Info2ActorState/MATLAB Function ==
  data: X input; Position output; Y input; Z input
function Position = fcn(X, Y, Z)

Position = [X Y, Z];

== matlab function ReqsGroundTruth/Vehicle Dynamics/Info2ActorState/MATLAB Function1 ==
  data: Xdot input; Velocity output; Ydot input; Zdot input
function Velocity = fcn(Xdot, Ydot, Zdot)

Velocity = [Xdot Ydot, Zdot];

== matlab function ReqsGroundTruth/Vehicle Dynamics/Info2ActorState/MATLAB Function2 ==
  data: aX input; Acceleration output; aY input; aZ input
function Acceleration = fcn(aX, aY, aZ)

Acceleration = [aX aY, aZ];

== matlab function ReqsGroundTruth/Vehicle Dynamics/Info2ActorState/MATLAB Function3 ==
  data: phiDot input; AngularVelocity output; thetaDot input; psiDot input
function AngularVelocity = fcn(phiDot, thetaDot, psiDot)

AngularVelocity = [phiDot thetaDot, psiDot];

== matlab function ReqsGroundTruth/Vehicle Dynamics/VehicleDynamics/engine-steer-brake dynamics/compute net torque ==
  data: gear input; Tnet output; Tengine input; Tbrake input; vc input
function Tnet  = net_torque(gear,Tengine,Tbrake,vc)

%  --set engine torque based on current gear selection

if (gear == 0)
    %  --vehicle is in PARK, so force engine torque to zero
    Tengine = 0;
end

Tnet = Tengine + Tbrake*tanh(5*vc);

end

== matlab function ReqsGroundTruth/Vehicle Dynamics/VehicleDynamics/engine-steer-brake dynamics/gear selection state machine ==
  data: gear output; gear_cmd input; vc input; Tbrake input; Tdead input; Vdead input
function gear = gear_change_FSM(gear_cmd,vc,Tbrake,Tdead,Vdead)

persistent GEAR

%  The vehicle gear can take on one of the following enumerated values:
%  -1 = REVERSE
%   0 = PARK
%   1 = DRIVE

%  --initialize the local persistent variables

if isempty(GEAR)
    %  --default gear at startup is PARK
    %  Note:  Change this to 1 if you want car to initialize in DRIVE
    GEAR = 0;
end


%  --evaluate the gear change finite state machine

switch GEAR
    case 0  % vehicle is in PARK
        if (gear_cmd == 1)
            %  --check to see if we can shift to DRIVE
            if ((abs(vc) <= Vdead) && (abs(Tbrake) > Tdead))
                %  --shift to DRIVE
                GEAR = 1;
            end
            
        elseif (gear_cmd == 2)
            %  --check to see if we can shift to REVERSE
            if ((abs(vc) <= Vdead) && (abs(Tbrake) > Tdead))
                %  --shift to REVERSE
                GEAR = 2;
            end
        end
        
    case 1  % vehicle is in DRIVE
        if (gear_cmd == 0)
            %  --check to see if we can shift to PARK
            if ((abs(vc) <= Vdead) && (abs(Tbrake) > Tdead))
                %  --shift to PARK
                GEAR = 0;
            end
            
        elseif (gear_cmd == 2)
            %  --check to see if we can shift to REVERSE
            if ((abs(vc) <= Vdead) && (abs(Tbrake) > Tdead))
                %  --shift to REVERSE
                GEAR = 2;
            end
        end
        
    case -1  % vehicle is in REVERSE
        if (gear_cmd == 0)
            %  --check to see if we can shift to PARK
            if ((abs(vc) <= Vdead) && (abs(Tbrake) > Tdead))
                %  --shift to PARK
                GEAR = 0;
            end
            
        elseif (gear_cmd == 1)
            %  --check to see if we can shift to DRIVE
            if ((abs(vc) <= Vdead) && (abs(Tbrake) > Tdead))
                %  --shift to DRIVE
                GEAR = 1;
            end
        end
        
    otherwise  %  --should never be here
        if (vc > Vdead)
            %  --moving forward, so must be in DRIVE
            GEAR = 1;
        elseif (vc < -Vdead)
            %  --moving backward, so must be in REVERSE
            GEAR = 2;
        else
            %  --vehicle stoppped, so must be in PARK
            GEAR = 0;
        end

end


%  --output the current actual gear setting

gear = GEAR;

return

== matlab function ReqsGroundTruth/Positions and States /MATLAB Function2 ==
  data: Actors input; ss_poses output; ss_State input

function ss_poses = findssposes(Actors, ss_State)

n=length(ss_State);
ss_poses=zeros(n,4);
indices=zeros(n,1);
ID=zeros(length(Actors),1);

for i=1:length(Actors)
 ID(i)=Actors(i).ActorID;
end

indices=find(ismember(ID,ss_State));
if(~isempty(indices))
    
    for i=1:n
        ss_poses(i,:)=([Actors(indices(i)).Position(:)',ss_State(i)]);
    end
end

ss_poses(ss_poses==0)=NaN;






% ss1_poses=zeros(1,4);
% ss2_poses=zeros(1,4);
% for i=1:length(Actors)
%     ID=Actors(i).ActorID;
%     
%     if(ID==ss1_State(1))
%         ss1_poses=[Actors(i).Position(:)',ss1_State(1)];
%     elseif ID== (ss1_State(2))
%         ss2_poses=[Actors(i).Position(:)',ss1_State(2)];
%     
%     end
%   
% end
% ss1_poses(ss1_poses==0)=NaN;   
% ss2_poses(ss2_poses==0)=NaN;

== matlab function ReqsGroundTruth/Positions and States /MATLAB Function1 ==
  data: Actors input; TL_poses output; TL_State input

function TL_poses = findTLposes(Actors, TL_State)
n=length(TL_State);
TL_poses=zeros(n/2,5);
indices=zeros(n/2,1);
ID=zeros(length(Actors),1);

for i=1:length(Actors)
 ID(i)=Actors(i).ActorID;
end

indices=find(ismember(ID,TL_State(n/2+1:end)));
if (~isempty(indices))

    for i=1:n/2
        TL_poses(i,:)=([Actors(indices(i)).Position(:)',TL_State(i),ID(indices(i))]);

    end
end
TL_poses(TL_poses==0)=NaN;

== stateflow chart ReqsGroundTruth/Positions and States /Traffic Light Sensor/Traffic Light Switching Logic ==
  state STEADYRED
    entry:
    trafficLight(:)= Red; TL_ID=TL_id;
  state STEADYGREEN
    entry:
    trafficLight(:)= Green; TL_ID=TL_id;
  state START
    entry:
    trafficLight=TL_id;
    trafficLight(:)= Black;TL_ID=TL_id;
  state TRAFFICLIGHT_ODDYELLOW_EVENRED
    entry:
    trafficLight(1:2:end)=Yellow;TL_ID(1:2:end)=TL_id(1:2:end);
    trafficLight(2:2:end) = Red;TL_ID(2:2:end)=TL_id(2:2:end);
  state TRAFFICLIGHT_ODDGREEN_EVENRED
    entry:
    trafficLight(1:2:end)=Green;TL_ID(1:2:end)=TL_id(1:2:end);
    trafficLight(2:2:end) = Red;TL_ID(2:2:end)=TL_id(2:2:end);
  state TRAFFICLIGHT_ODDRED_EVENYELLOW
    entry:
    trafficLight(1:2:end)=Red;TL_ID(1:2:end)=TL_id(1:2:end);
    trafficLight(2:2:end) = Yellow;TL_ID(2:2:end)=TL_id(2:2:end);
  state TRAFFICLIGHT_ODDRED_EVENGREEN
    entry:
    trafficLight(1:2:end)=Red;TL_ID(1:2:end)=TL_id(1:2:end);
    trafficLight(2:2:end) = Green;TL_ID(2:2:end)=TL_id(2:2:end);
  (default) -> START
  START -> STEADYGREEN [order 3] : [LightConfig==1]
  START -> STEADYRED [order 1] : [LightConfig==2]
  START -> TRAFFICLIGHT_ODDGREEN_EVENRED [order 2] : [LightConfig ==3]
  TRAFFICLIGHT_ODDGREEN_EVENRED -> TRAFFICLIGHT_ODDYELLOW_EVENRED : after(0.5,sec)
  TRAFFICLIGHT_ODDYELLOW_EVENRED -> TRAFFICLIGHT_ODDRED_EVENGREEN : after(0.5,sec)
  TRAFFICLIGHT_ODDRED_EVENYELLOW -> TRAFFICLIGHT_ODDGREEN_EVENRED : after(0.5,sec)
  TRAFFICLIGHT_ODDRED_EVENGREEN -> TRAFFICLIGHT_ODDRED_EVENYELLOW : after(0.5,sec)
  data: Green constant double =3; Red constant double =1; Yellow constant double =2; LightConfig input; TL_id input; Black constant double =0; TL_ID output; trafficLight output
